simulink library "lib_controller"  (R2015a)
settings: Solver=ode45  StartTime=0.0  StopTime=10.0  RelTol=1e-3
values from neighbouring files (symbols this model uses):
  CG_0 = [0,0,0.02]'    [SetupComplete.m]
  g = 9.81    [SetupComplete.m]
  h_M = 0.064    [SetupComplete.m]
  I_BAC_0 = [ Ix,0,Ixz;0,Iy,0;Ixz,0,Iz]    [SetupComplete.m]
  l = 0.3450    (= 0.345)    [NDI_components.m]    (also in SetupComplete.m; robust_controller.m)
  m = 3.51    [SetupComplete.m]
  m_0 = 2.61    [SetupComplete.m]
  m_M = 0.300    (= 0.3)    [SetupComplete.m]
  T_sim = 0.01    [Run3Copter.m]
undefined symbols (not defined in the file or in its folder): Theta_1_roll_last, Theta_2_roll_last, Theta_3_roll_last, V_long_lastA_w_z, V_long_lastAoA, V_roll_last, V_yaw_last, W_long_lastA_w_z, W_long_lastAoA, W_roll_last, W_yaw_last
libraries: simulink x65, Adaptive_FaultTolerantControl x8, lib_controller x5, qcatlib x4, dspinverses x4, aerolibtransform2 x3, aerolib6dofsys x1
(part 8 of 10)

== matlab function lib_controller/Controller/NDI+CA Controller/4DOF NDI+CA Controller/F(X)1 ==
  data: I_BAC input; CG input; gx output; prev_input input
function gx = gx(I_BAC, CG, prev_input)
    % Calculates f_hat(x). The expression is calculated in NDI_components
    % x_dot = f(x) + g(x,u)
    %   g(x,u) ~= g(x,u0) + jac(g(x,u), u)(u0) * (u - u0)
    %   g(x,u) ~= h(x,u0) + jac(g(x,u), u)(u0) * u
    % x_dot = f_hat(x) + jac(g(x,u), u) * u
    %   f_hat(x) = f(x) + g(x,u0) - jac(g(x,u), u)(u0) *  u0
    %   g_hat(x) = jac(g(x,u), u)(u0)
    % x_dot = f_hat(x) + g_hat(x) * u
    Ixx = I_BAC(1,1);
    Iyy = I_BAC(2,2);
    Izz = I_BAC(3,3);
    Ixz = I_BAC(1,3);
    Iyz = I_BAC(2,3);
    cx = CG(1);
    cy = CG(2);
    cz = CG(3);
    tau1_0 = prev_input(1);
    eta1_0 = prev_input(2);
    gamma1_0 = prev_input(3);
    tau2_0 = prev_input(4);
    eta2_0 = prev_input(5);
    gamma2_0 = prev_input(6);
    tau3_0 = prev_input(7);
    eta3_0 = prev_input(8);
    gamma3_0 = prev_input(9);

 gx = [...
     
                                                                                                                                                                                                                                                                                                                                                         (Gx*Ixx*Iyz^2 + Gx*Ixz^2*Iyy + Gx*Ixy^2*Izz + 2*Gx*Ixy*Ixz*Iyz - Gx*Ixx*Iyy*Izz + Ixy^3*P^2*cy*mass + Ixz^3*P^2*cz*mass - Ixy^3*Q^2*cy*mass - Ixz^3*R^2*cz*mass - Ixx*Iyz^2*Q*W*mass + Ixx*Iyz^2*R*V*mass - Ixz^2*Iyy*Q*W*mass + Ixz^2*Iyy*R*V*mass - Ixy^2*Izz*Q*W*mass + Ixy^2*Izz*R*V*mass + Ixy*Ixz^2*P^2*cy*mass + Ixy^2*Ixz*P^2*cz*mass + Ixx*Iyz^2*Q^2*cx*mass + Ixz^2*Iyy*Q^2*cx*mass - Ixy*Iyz^2*Q^2*cy*mass - Ixy^2*Ixz*Q^2*cz*mass + Ixy^2*Izz*Q^2*cx*mass + Ixz*Iyz^2*Q^2*cz*mass + Ixx*Iyz^2*R^2*cx*mass - Ixy*Ixz^2*R^2*cy*mass + Ixz^2*Iyy*R^2*cx*mass + Ixy*Iyz^2*R^2*cy*mass + Ixy^2*Izz*R^2*cx*mass - Ixz*Iyz^2*R^2*cz*mass + Ixx*Iyz^2*Kt*gamma1_0*tau1_0*cos(gamma1_0) + Ixz^2*Iyy*Kt*gamma1_0*tau1_0*cos(gamma1_0) + Ixy^2*Izz*Kt*gamma1_0*tau1_0*cos(gamma1_0) - 2*Ixy*Ixz*Iyz*Q*W*mass + 2*Ixy*Ixz*Iyz*R*V*mass + Ixx*Iyy*Izz*Q*W*mass - Ixx*Iyy*Izz*R*V*mass - Ixx*Ixy*Iyy*P^2*cy*mass + Ixx*Ixz*Iyz*P^2*cy*mass + Ixx*Ixy*Iyz*P^2*cz*mass - Ixx*Ixz*Izz*P^2*cz*mass + 2*Ixy*Ixz*Iyz*Q^2*cx*mass + Ixx*Ixy*Iyy*Q^2*cy*mass - Ixx*Ixy*Iyz*Q^2*cz*mass - Ixx*Iyy*Izz*Q^2*cx*mass - Ixz*Iyy*Iyz*Q^2*cy*mass + Ixy*Iyz*Izz*Q^2*cz*mass + 2*Ixy*Ixz*Iyz*R^2*cx*mass - Ixx*Ixz*Iyz*R^2*cy*mass - Ixx*Iyy*Izz*R^2*cx*mass + Ixz*Iyy*Iyz*R^2*cy*mass + Ixx*Ixz*Izz*R^2*cz*mass - Ixy*Iyz*Izz*R^2*cz*mass + Ixx*Ixy^2*P*Q*cy*mass + Ixx*Iyy^2*P*Q*cy*mass - Ixx^2*Iyy*P*Q*cy*mass - Ixy^2*Iyy*P*Q*cy*mass - 2*Ixz^2*Iyy*P*Q*cy*mass + Ixx^2*Iyz*P*Q*cz*mass - Ixy^2*Izz*P*Q*cy*mass + 2*Ixz^2*Iyz*P*Q*cz*mass + Ixx*Ixz^2*P*R*cz*mass + Ixx^2*Iyz*P*R*cy*mass + 2*Ixy^2*Iyz*P*R*cy*mass - Ixz^2*Iyy*P*R*cz*mass + Ixx*Izz^2*P*R*cz*mass - Ixx^2*Izz*P*R*cz*mass - 2*Ixy^2*Izz*P*R*cz*mass - Ixz^2*Izz*P*R*cz*mass - 2*Ixy^2*Ixz*Q*R*cy*mass - 2*Ixy*Ixz^2*Q*R*cz*mass - Ixz*Iyy^2*Q*R*cy*mass - Ixy*Izz^2*Q*R*cz*mass + Ixx*Iyz^2*Kt*eta2_0*tau2_0*cos(eta2_0)*cos(gamma2_0) + Ixx*Iyz^2*Kt*eta3_0*tau3_0*cos(eta3_0)*cos(gamma3_0) + Ixz^2*Iyy*Kt*eta2_0*tau2_0*cos(eta2_0)*cos(gamma2_0) + Ixz^2*Iyy*Kt*eta3_0*tau3_0*cos(eta3_0)*cos(gamma3_0) + Ixy^2*Izz*Kt*eta2_0*tau2_0*cos(eta2_0)*cos(gamma2_0) + Ixy^2*Izz*Kt*eta3_0*tau3_0*cos(eta3_0)*cos(gamma3_0) - Ixx*Iyz^2*Kt*gamma2_0*tau2_0*sin(eta2_0)*sin(gamma2_0) - Ixx*Iyz^2*Kt*gamma3_0*tau3_0*sin(eta3_0)*sin(gamma3_0) - Ixz^2*Iyy*Kt*gamma2_0*tau2_0*sin(eta2_0)*sin(gamma2_0) - Ixz^2*Iyy*Kt*gamma3_0*tau3_0*sin(eta3_0)*sin(gamma3_0) - Ixy^2*Izz*Kt*gamma2_0*tau2_0*sin(eta2_0)*sin(gamma2_0) - Ixy^2*Izz*Kt*gamma3_0*tau3_0*sin(eta3_0)*sin(gamma3_0) + 2*Ixy*Ixz*Iyz*Kt*gamma1_0*tau1_0*cos(gamma1_0) - Ixx*Iyy*Izz*Kt*gamma1_0*tau1_0*cos(gamma1_0) + Ixx*Ixy*Ixz*P*Q*cz*mass - 2*Ixy*Ixz*Iyz*P*Q*cy*mass - Ixy*Ixz*Iyy*P*Q*cz*mass - Ixx*Iyy*Iyz*P*Q*cz*mass + Ixx*Iyy*Izz*P*Q*cy*mass + Ixy*Ixz*Izz*P*Q*cz*mass - Ixx*Iyz*Izz*P*Q*cz*mass + Ixx*Ixy*Ixz*P*R*cy*mass + Ixy*Ixz*Iyy*P*R*cy*mass - Ixx*Iyy*Iyz*P*R*cy*mass - 2*Ixy*Ixz*Iyz*P*R*cz*mass - Ixy*Ixz*Izz*P*R*cy*mass - Ixx*Iyz*Izz*P*R*cy*mass + Ixx*Iyy*Izz*P*R*cz*mass - Ixx*Ixy*Iyz*Q*R*cy*mass + Ixx*Ixz*Iyy*Q*R*cy*mass - Ixx*Ixz*Iyz*Q*R*cz*mass - Ixy*Iyy*Iyz*Q*R*cy*mass + Ixx*Ixy*Izz*Q*R*cz*mass + Ixy*Iyz*Izz*Q*R*cy*mass + Ixz*Iyy*Iyz*Q*R*cz*mass + Ixz*Iyy*Izz*Q*R*cy*mass + Ixy*Iyy*Izz*Q*R*cz*mass - Ixz*Iyz*Izz*Q*R*cz*mass - Ixz^2*Kq*cz*gamma2_0*mass*tau2_0*cos(gamma2_0) - Ixz^2*Kq*cz*gamma3_0*mass*tau3_0*cos(gamma3_0) - 2*Ixy*Ixz*Iyz*Kt*gamma2_0*tau2_0*sin(eta2_0)*sin(gamma2_0) - 2*Ixy*Ixz*Iyz*Kt*gamma3_0*tau3_0*sin(eta3_0)*sin(gamma3_0) + Ixx*Iyy*Izz*Kt*gamma2_0*tau2_0*sin(eta2_0)*sin(gamma2_0) + Ixx*Iyy*Izz*Kt*gamma3_0*tau3_0*sin(eta3_0)*sin(gamma3_0) + Ixz^2*Kq*cz*eta1_0*mass*tau1_0*cos(eta1_0)*cos(gamma1_0) - Ixy^2*Kq*cy*eta1_0*mass*tau1_0*cos(gamma1_0)*sin(eta1_0) + Ixy^2*Kq*cy*eta2_0*mass*tau2_0*cos(gamma2_0)*sin(eta2_0) + Ixy^2*Kq*cy*eta3_0*mass*tau3_0*cos(gamma3_0)*sin(eta3_0) - Ixy^2*Kq*cy*gamma1_0*mass*tau1_0*cos(eta1_0)*sin(gamma1_0) + Ixy^2*Kq*cy*gamma2_0*mass*tau2_0*cos(eta2_0)*sin(gamma2_0) + Ixy^2*Kq*cy*gamma3_0*mass*tau3_0*cos(eta3_0)*sin(gamma3_0) - Ixz^2*Kq*cz*gamma1_0*mass*tau1_0*sin(eta1_0)*sin(gamma1_0) - Ixy*Ixz*Kq*cy*gamma2_0*mass*tau2_0*cos(gamma2_0) - Ixy*Ixz*Kq*cy*gamma3_0*mass*tau3_0*cos(gamma3_0) - Ixx*Iyz*Kq*cy*gamma2_0*mass*tau2_0*cos(gamma2_0) - Ixx*Iyz*Kq*cy*gamma3_0*mass*tau3_0*cos(gamma3_0) - Ixy*Iyz*Kq*cy*gamma1_0*mass*tau1_0*cos(gamma1_0) - Ixz*Iyy*Kq*cy*gamma1_0*mass*tau1_0*cos(gamma1_0) + Ixz*Iyz*Kq*cz*gamma1_0*mass*tau1_0*cos(gamma1_0) + Ixx*Izz*Kq*cz*gamma2_0*mass*tau2_0*cos(gamma2_0) + Ixx*Izz*Kq*cz*gamma3_0*mass*tau3_0*cos(gamma3_0) + Ixy*Izz*Kq*cz*gamma1_0*mass*tau1_0*cos(gamma1_0) + 2*Ixy*Ixz*Iyz*Kt*eta2_0*tau2_0*cos(eta2_0)*cos(gamma2_0) + 2*Ixy*Ixz*Iyz*Kt*eta3_0*tau3_0*cos(eta3_0)*cos(gamma3_0) - Ixx*Iyy*Izz*Kt*eta2_0*tau2_0*cos(eta2_0)*cos(gamma2_0) - Ixx*Iyy*Izz*Kt*eta3_0*tau3_0*cos(eta3_0)*cos(gamma3_0) + Ixy*Ixz*Kq*cy*eta1_0*mass*tau1_0*cos(eta1_0)*cos(gamma1_0) + Ixx*Iyz*Kq*cy*eta1_0*mass*tau1_0*cos(eta1_0)*cos(gamma1_0) + Ixy*Iyz*Kq*cy*eta2_0*mass*tau2_0*cos(eta2_0)*cos(gamma2_0) + Ixz*Iyy*Kq*cy*eta2_0*mass*tau2_0*cos(eta2_0)*cos(gamma2_0) + Ixy*Iyz*Kq*cy*eta3_0*mass*tau3_0*cos(eta3_0)*cos(gamma3_0) + Ixz*Iyy*Kq*cy*eta3_0*mass*tau3_0*cos(eta3_0)*cos(gamma3_0) - Ixz*Iyz*Kq*cz*eta2_0*mass*tau2_0*cos(eta2_0)*cos(gamma2_0) - Ixz*Iyz*Kq*cz*eta3_0*mass*tau3_0*cos(eta3_0)*cos(gamma3_0) - Ixx*Izz*Kq*cz*eta1_0*mass*tau1_0*cos(eta1_0)*cos(gamma1_0) - Ixy*Izz*Kq*cz*eta2_0*mass*tau2_0*cos(eta2_0)*cos(gamma2_0) - Ixy*Izz*Kq*cz*eta3_0*mass*tau3_0*cos(eta3_0)*cos(gamma3_0) + Ixx*Iyy*Kq*cy*eta1_0*mass*tau1_0*cos(gamma1_0)*sin(eta1_0) - Ixx*Iyy*Kq*cy*eta2_0*mass*tau2_0*cos(gamma2_0)*sin(eta2_0) - Ixx*Iyy*Kq*cy*eta3_0*mass*tau3_0*cos(gamma3_0)*sin(eta3_0) - Ixy*Ixz*Kq*cz*eta1_0*mass*tau1_0*cos(gamma1_0)*sin(eta1_0) + Ixy*Ixz*Kq*cz*eta2_0*mass*tau2_0*cos(gamma2_0)*sin(eta2_0) + Ixy*Ixz*Kq*cz*eta3_0*mass*tau3_0*cos(gamma3_0)*sin(eta3_0) - Ixx*Iyz*Kq*cz*eta1_0*mass*tau1_0*cos(gamma1_0)*sin(eta1_0) + Ixx*Iyz*Kq*cz*eta2_0*mass*tau2_0*cos(gamma2_0)*sin(eta2_0) + Ixx*Iyz*Kq*cz*eta3_0*mass*tau3_0*cos(gamma3_0)*sin(eta3_0) + Ixx*Iyy*Kq*cy*gamma1_0*mass*tau1_0*cos(eta1_0)*sin(gamma1_0) - Ixx*Iyy*Kq*cy*gamma2_0*mass*tau2_0*cos(eta2_0)*sin(gamma2_0) - Ixx*Iyy*Kq*cy*gamma3_0*mass*tau3_0*cos(eta3_0)*sin(gamma3_0) - Ixy*Ixz*Kq*cz*gamma1_0*mass*tau1_0*cos(eta1_0)*sin(gamma1_0) + Ixy*Ixz*Kq*cz*gamma2_0*mass*tau2_0*cos(eta2_0)*sin(gamma2_0) + Ixy*Ixz*Kq*cz*gamma3_0*mass*tau3_0*cos(eta3_0)*sin(gamma3_0) - Ixx*Iyz*Kq*cz*gamma1_0*mass*tau1_0*cos(eta1_0)*sin(gamma1_0) + Ixx*Iyz*Kq*cz*gamma2_0*mass*tau2_0*cos(eta2_0)*sin(gamma2_0) + Ixx*Iyz*Kq*cz*gamma3_0*mass*tau3_0*cos(eta3_0)*sin(gamma3_0) - Ixy*Ixz*Kq*cy*gamma1_0*mass*tau1_0*sin(eta1_0)*sin(gamma1_0) - Ixx*Iyz*Kq*cy*gamma1_0*mass*tau1_0*sin(eta1_0)*sin(gamma1_0) - Ixy*Iyz*Kq*cy*gamma2_0*mass*tau2_0*sin(eta2_0)*sin(gamma2_0) - Ixz*Iyy*Kq*cy*gamma2_0*mass*tau2_0*sin(eta2_0)*sin(gamma2_0) - Ixy*Iyz*Kq*cy*gamma3_0*mass*tau3_0*sin(eta3_0)*sin(gamma3_0) - Ixz*Iyy*Kq*cy*gamma3_0*mass*tau3_0*sin(eta3_0)*sin(gamma3_0) + Ixz*Iyz*Kq*cz*gamma2_0*mass*tau2_0*sin(eta2_0)*sin(gamma2_0) + Ixz*Iyz*Kq*cz*gamma3_0*mass*tau3_0*sin(eta3_0)*sin(gamma3_0) + Ixx*Izz*Kq*cz*gamma1_0*mass*tau1_0*sin(eta1_0)*sin(gamma1_0) + Ixy*Izz*Kq*cz*gamma2_0*mass*tau2_0*sin(eta2_0)*sin(gamma2_0) + Ixy*Izz*Kq*cz*gamma3_0*mass*tau3_0*sin(eta3_0)*sin(gamma3_0))/(mass*(Izz*Ixy^2 + 2*Ixy*Ixz*Iyz + Iyy*Ixz^2 + Ixx*Iyz^2 - Ixx*Iyy*Izz));
                                                                                                                                                                                                                                                                                                                                                                                                                                                                                                                                                                                                                                                                                                               -(Gy*Ixx*Iyy*Izz - Gy*Ixz^2*Iyy - Gy*Ixy^2*Izz - 2*Gy*Ixy*Ixz*Iyz - Gy*Ixx*Iyz^2 + Ixy^3*P^2*cx*mass - Ixy^3*Q^2*cx*mass - Iyz^3*Q^2*cz*mass + Iyz^3*R^2*cz*mass - Ixx*Iyz^2*P*W*mass + Ixx*Iyz^2*R*U*mass - Ixz^2*Iyy*P*W*mass + Ixz^2*Iyy*R*U*mass - Ixy^2*Izz*P*W*mass + Ixy^2*Izz*R*U*mass + Ixy*Ixz^2*P^2*cx*mass - Ixx*Iyz^2*P^2*cy*mass - Ixz^2*Iyy*P^2*cy*mass + Ixy^2*Iyz*P^2*cz*mass - Ixy^2*Izz*P^2*cy*mass - Ixz^2*Iyz*P^2*cz*mass - Ixy*Iyz^2*Q^2*cx*mass - Ixy^2*Iyz*Q^2*cz*mass - Ixy*Ixz^2*R^2*cx*mass + Ixy*Iyz^2*R^2*cx*mass - Ixx*Iyz^2*R^2*cy*mass - Ixz^2*Iyy*R^2*cy*mass - Ixy^2*Izz*R^2*cy*mass + Ixz^2*Iyz*R^2*cz*mass + Ixx*Iyz^2*Kt*gamma2_0*tau2_0*cos(gamma2_0) + Ixx*Iyz^2*Kt*gamma3_0*tau3_0*cos(gamma3_0) + Ixz^2*Iyy*Kt*gamma2_0*tau2_0*cos(gamma2_0) + Ixz^2*Iyy*Kt*gamma3_0*tau3_0*cos(gamma3_0) + Ixy^2*Izz*Kt*gamma2_0*tau2_0*cos(gamma2_0) + Ixy^2*Izz*Kt*gamma3_0*tau3_0*cos(gamma3_0) - 2*Ixy*Ixz*Iyz*P*W*mass + 2*Ixy*Ixz*Iyz*R*U*mass + Ixx*Iyy*Izz*P*W*mass - Ixx*Iyy*Izz*R*U*mass - Ixx*Ixy*Iyy*P^2*cx*mass + Ixx*Ixz*Iyz*P^2*cx*mass - 2*Ixy*Ixz*Iyz*P^2*cy*mass + Ixy*Ixz*Iyy*P^2*cz*mass + Ixx*Iyy*Izz*P^2*cy*mass - Ixy*Ixz*Izz*P^2*cz*mass + Ixx*Ixy*Iyy*Q^2*cx*mass - Ixz*Iyy*Iyz*Q^2*cx*mass - Ixy*Ixz*Iyy*Q^2*cz*mass + Iyy*Iyz*Izz*Q^2*cz*mass - Ixx*Ixz*Iyz*R^2*cx*mass - 2*Ixy*Ixz*Iyz*R^2*cy*mass + Ixz*Iyy*Iyz*R^2*cx*mass + Ixx*Iyy*Izz*R^2*cy*mass + Ixy*Ixz*Izz*R^2*cz*mass - Iyy*Iyz*Izz*R^2*cz*mass + Ixx*Ixy^2*P*Q*cx*mass + Ixx*Iyy^2*P*Q*cx*mass - Ixx^2*Iyy*P*Q*cx*mass + 2*Ixx*Iyz^2*P*Q*cx*mass - Ixy^2*Iyy*P*Q*cx*mass + Ixy^2*Izz*P*Q*cx*mass - Ixz*Iyy^2*P*Q*cz*mass - 2*Ixz*Iyz^2*P*Q*cz*mass + Ixx^2*Iyz*P*R*cx*mass + 2*Ixy^2*Iyz*P*R*cx*mass + 2*Ixy*Iyz^2*P*R*cz*mass + Ixy*Izz^2*P*R*cz*mass - 2*Ixy^2*Ixz*Q*R*cx*mass - Ixz*Iyy^2*Q*R*cx*mass + Ixx*Iyz^2*Q*R*cz*mass - Iyy*Iyz^2*Q*R*cz*mass + 2*Ixy^2*Izz*Q*R*cz*mass - Iyy*Izz^2*Q*R*cz*mass + Iyy^2*Izz*Q*R*cz*mass + Iyz^2*Izz*Q*R*cz*mass + Ixx*Iyz^2*Kt*eta1_0*tau1_0*cos(eta1_0)*cos(gamma1_0) + Ixz^2*Iyy*Kt*eta1_0*tau1_0*cos(eta1_0)*cos(gamma1_0) + Ixy^2*Izz*Kt*eta1_0*tau1_0*cos(eta1_0)*cos(gamma1_0) - Ixx*Iyz^2*Kt*gamma1_0*tau1_0*sin(eta1_0)*sin(gamma1_0) - Ixz^2*Iyy*Kt*gamma1_0*tau1_0*sin(eta1_0)*sin(gamma1_0) - Ixy^2*Izz*Kt*gamma1_0*tau1_0*sin(eta1_0)*sin(gamma1_0) + 2*Ixy*Ixz*Iyz*Kt*gamma2_0*tau2_0*cos(gamma2_0) + 2*Ixy*Ixz*Iyz*Kt*gamma3_0*tau3_0*cos(gamma3_0) - Ixx*Iyy*Izz*Kt*gamma2_0*tau2_0*cos(gamma2_0) - Ixx*Iyy*Izz*Kt*gamma3_0*tau3_0*cos(gamma3_0) + 2*Ixy*Ixz*Iyz*P*Q*cx*mass + Ixx*Ixy*Iyz*P*Q*cz*mass + Ixx*Ixz*Iyy*P*Q*cz*mass - Ixx*Iyy*Izz*P*Q*cx*mass - Ixy*Iyy*Iyz*P*Q*cz*mass - Ixy*Iyz*Izz*P*Q*cz*mass + Ixz*Iyy*Izz*P*Q*cz*mass + Ixx*Ixy*Ixz*P*R*cx*mass + Ixy*Ixz*Iyy*P*R*cx*mass - Ixx*Iyy*Iyz*P*R*cx*mass - Ixy*Ixz*Izz*P*R*cx*mass - Ixx*Ixz*Iyz*P*R*cz*mass - Ixx*Iyz*Izz*P*R*cx*mass - Ixx*Ixy*Izz*P*R*cz*mass + Ixz*Iyy*Iyz*P*R*cz*mass - Ixy*Iyy*Izz*P*R*cz*mass + Ixz*Iyz*Izz*P*R*cz*mass - Ixx*Ixy*Iyz*Q*R*cx*mass + Ixx*Ixz*Iyy*Q*R*cx*mass - Ixy*Iyy*Iyz*Q*R*cx*mass + 2*Ixy*Ixz*Iyz*Q*R*cz*mass + Ixy*Iyz*Izz*Q*R*cx*mass + Ixz*Iyy*Izz*Q*R*cx*mass - Ixx*Iyy*Izz*Q*R*cz*mass - Iyz^2*Kq*cz*gamma1_0*mass*tau1_0*cos(gamma1_0) - 2*Ixy*Ixz*Iyz*Kt*gamma1_0*tau1_0*sin(eta1_0)*sin(gamma1_0) + Ixx*Iyy*Izz*Kt*gamma1_0*tau1_0*sin(eta1_0)*sin(gamma1_0) + Iyz^2*Kq*cz*eta2_0*mass*tau2_0*cos(eta2_0)*cos(gamma2_0) + Iyz^2*Kq*cz*eta3_0*mass*tau3_0*cos(eta3_0)*cos(gamma3_0) - Ixy^2*Kq*cx*eta1_0*mass*tau1_0*cos(gamma1_0)*sin(eta1_0) + Ixy^2*Kq*cx*eta2_0*mass*tau2_0*cos(gamma2_0)*sin(eta2_0) + Ixy^2*Kq*cx*eta3_0*mass*tau3_0*cos(gamma3_0)*sin(eta3_0) - Ixy^2*Kq*cx*gamma1_0*mass*tau1_0*cos(eta1_0)*sin(gamma1_0) + Ixy^2*Kq*cx*gamma2_0*mass*tau2_0*cos(eta2_0)*sin(gamma2_0) + Ixy^2*Kq*cx*gamma3_0*mass*tau3_0*cos(eta3_0)*sin(gamma3_0) - Iyz^2*Kq*cz*gamma2_0*mass*tau2_0*sin(eta2_0)*sin(gamma2_0) - Iyz^2*Kq*cz*gamma3_0*mass*tau3_0*sin(eta3_0)*sin(gamma3_0) - Ixy*Ixz*Kq*cx*gamma2_0*mass*tau2_0*cos(gamma2_0) - Ixy*Ixz*Kq*cx*gamma3_0*mass*tau3_0*cos(gamma3_0) - Ixx*Iyz*Kq*cx*gamma2_0*mass*tau2_0*cos(gamma2_0) - Ixx*Iyz*Kq*cx*gamma3_0*mass*tau3_0*cos(gamma3_0) - Ixy*Iyz*Kq*cx*gamma1_0*mass*tau1_0*cos(gamma1_0) - Ixz*Iyy*Kq*cx*gamma1_0*mass*tau1_0*cos(gamma1_0) + Ixz*Iyz*Kq*cz*gamma2_0*mass*tau2_0*cos(gamma2_0) + Ixz*Iyz*Kq*cz*gamma3_0*mass*tau3_0*cos(gamma3_0) + Ixy*Izz*Kq*cz*gamma2_0*mass*tau2_0*cos(gamma2_0) + Ixy*Izz*Kq*cz*gamma3_0*mass*tau3_0*cos(gamma3_0) + Iyy*Izz*Kq*cz*gamma1_0*mass*tau1_0*cos(gamma1_0) + 2*Ixy*Ixz*Iyz*Kt*eta1_0*tau1_0*cos(eta1_0)*cos(gamma1_0) - Ixx*Iyy*Izz*Kt*eta1_0*tau1_0*cos(eta1_0)*cos(gamma1_0) + Ixy*Ixz*Kq*cx*eta1_0*mass*tau1_0*cos(eta1_0)*cos(gamma1_0) + Ixx*Iyz*Kq*cx*eta1_0*mass*tau1_0*cos(eta1_0)*cos(gamma1_0) + Ixy*Iyz*Kq*cx*eta2_0*mass*tau2_0*cos(eta2_0)*cos(gamma2_0) + Ixz*Iyy*Kq*cx*eta2_0*mass*tau2_0*cos(eta2_0)*cos(gamma2_0) + Ixy*Iyz*Kq*cx*eta3_0*mass*tau3_0*cos(eta3_0)*cos(gamma3_0) + Ixz*Iyy*Kq*cx*eta3_0*mass*tau3_0*cos(eta3_0)*cos(gamma3_0) - Ixz*Iyz*Kq*cz*eta1_0*mass*tau1_0*cos(eta1_0)*cos(gamma1_0) - Ixy*Izz*Kq*cz*eta1_0*mass*tau1_0*cos(eta1_0)*cos(gamma1_0) - Iyy*Izz*Kq*cz*eta2_0*mass*tau2_0*cos(eta2_0)*cos(gamma2_0) - Iyy*Izz*Kq*cz*eta3_0*mass*tau3_0*cos(eta3_0)*cos(gamma3_0) + Ixx*Iyy*Kq*cx*eta1_0*mass*tau1_0*cos(gamma1_0)*sin(eta1_0) - Ixx*Iyy*Kq*cx*eta2_0*mass*tau2_0*cos(gamma2_0)*sin(eta2_0) - Ixx*Iyy*Kq*cx*eta3_0*mass*tau3_0*cos(gamma3_0)*sin(eta3_0) - Ixy*Iyz*Kq*cz*eta1_0*mass*tau1_0*cos(gamma1_0)*sin(eta1_0) - Ixz*Iyy*Kq*cz*eta1_0*mass*tau1_0*cos(gamma1_0)*sin(eta1_0) + Ixy*Iyz*Kq*cz*eta2_0*mass*tau2_0*cos(gamma2_0)*sin(eta2_0) + Ixz*Iyy*Kq*cz*eta2_0*mass*tau2_0*cos(gamma2_0)*sin(eta2_0) + Ixy*Iyz*Kq*cz*eta3_0*mass*tau3_0*cos(gamma3_0)*sin(eta3_0) + Ixz*Iyy*Kq*cz*eta3_0*mass*tau3_0*cos(gamma3_0)*sin(eta3_0) + Ixx*Iyy*Kq*cx*gamma1_0*mass*tau1_0*cos(eta1_0)*sin(gamma1_0) - Ixx*Iyy*Kq*cx*gamma2_0*mass*tau2_0*cos(eta2_0)*sin(gamma2_0) - Ixx*Iyy*Kq*cx*gamma3_0*mass*tau3_0*cos(eta3_0)*sin(gamma3_0) - Ixy*Iyz*Kq*cz*gamma1_0*mass*tau1_0*cos(eta1_0)*sin(gamma1_0) - Ixz*Iyy*Kq*cz*gamma1_0*mass*tau1_0*cos(eta1_0)*sin(gamma1_0) + Ixy*Iyz*Kq*cz*gamma2_0*mass*tau2_0*cos(eta2_0)*sin(gamma2_0) + Ixz*Iyy*Kq*cz*gamma2_0*mass*tau2_0*cos(eta2_0)*sin(gamma2_0) + Ixy*Iyz*Kq*cz*gamma3_0*mass*tau3_0*cos(eta3_0)*sin(gamma3_0) + Ixz*Iyy*Kq*cz*gamma3_0*mass*tau3_0*cos(eta3_0)*sin(gamma3_0) - Ixy*Ixz*Kq*cx*gamma1_0*mass*tau1_0*sin(eta1_0)*sin(gamma1_0) - Ixx*Iyz*Kq*cx*gamma1_0*mass*tau1_0*sin(eta1_0)*sin(gamma1_0) - Ixy*Iyz*Kq*cx*gamma2_0*mass*tau2_0*sin(eta2_0)*sin(gamma2_0) - Ixz*Iyy*Kq*cx*gamma2_0*mass*tau2_0*sin(eta2_0)*sin(gamma2_0) - Ixy*Iyz*Kq*cx*gamma3_0*mass*tau3_0*sin(eta3_0)*sin(gamma3_0) - Ixz*Iyy*Kq*cx*gamma3_0*mass*tau3_0*sin(eta3_0)*sin(gamma3_0) + Ixz*Iyz*Kq*cz*gamma1_0*mass*tau1_0*sin(eta1_0)*sin(gamma1_0) + Ixy*Izz*Kq*cz*gamma1_0*mass*tau1_0*sin(eta1_0)*sin(gamma1_0) + Iyy*Izz*Kq*cz*gamma2_0*mass*tau2_0*sin(eta2_0)*sin(gamma2_0) + Iyy*Izz*Kq*cz*gamma3_0*mass*tau3_0*sin(eta3_0)*sin(gamma3_0))/(mass*(Izz*Ixy^2 + 2*Ixy*Ixz*Iyz + Iyy*Ixz^2 + Ixx*Iyz^2 - Ixx*Iyy*Izz));
 -(Gz*Ixx*Iyy*Izz - Gz*Ixz^2*Iyy - Gz*Ixy^2*Izz - 2*Gz*Ixy*Ixz*Iyz - Gz*Ixx*Iyz^2 + Ixz^3*P^2*cx*mass + Iyz^3*Q^2*cy*mass - Ixz^3*R^2*cx*mass - Iyz^3*R^2*cy*mass + Ixx*Iyz^2*P*V*mass - Ixx*Iyz^2*Q*U*mass + Ixz^2*Iyy*P*V*mass - Ixz^2*Iyy*Q*U*mass + Ixy^2*Izz*P*V*mass - Ixy^2*Izz*Q*U*mass + Ixy^2*Ixz*P^2*cx*mass - Ixy^2*Iyz*P^2*cy*mass + Ixz^2*Iyz*P^2*cy*mass - Ixx*Iyz^2*P^2*cz*mass - Ixz^2*Iyy*P^2*cz*mass - Ixy^2*Izz*P^2*cz*mass - Ixy^2*Ixz*Q^2*cx*mass + Ixz*Iyz^2*Q^2*cx*mass + Ixy^2*Iyz*Q^2*cy*mass - Ixx*Iyz^2*Q^2*cz*mass - Ixz^2*Iyy*Q^2*cz*mass - Ixy^2*Izz*Q^2*cz*mass - Ixz*Iyz^2*R^2*cx*mass - Ixz^2*Iyz*R^2*cy*mass + 2*Ixy*Ixz*Iyz*P*V*mass - 2*Ixy*Ixz*Iyz*Q*U*mass - Ixx*Iyy*Izz*P*V*mass + Ixx*Iyy*Izz*Q*U*mass + Ixx*Ixy*Iyz*P^2*cx*mass - Ixx*Ixz*Izz*P^2*cx*mass - Ixy*Ixz*Iyy*P^2*cy*mass - 2*Ixy*Ixz*Iyz*P^2*cz*mass + Ixy*Ixz*Izz*P^2*cy*mass + Ixx*Iyy*Izz*P^2*cz*mass - Ixx*Ixy*Iyz*Q^2*cx*mass + Ixy*Ixz*Iyy*Q^2*cy*mass - 2*Ixy*Ixz*Iyz*Q^2*cz*mass + Ixy*Iyz*Izz*Q^2*cx*mass + Ixx*Iyy*Izz*Q^2*cz*mass - Iyy*Iyz*Izz*Q^2*cy*mass + Ixx*Ixz*Izz*R^2*cx*mass - Ixy*Ixz*Izz*R^2*cy*mass - Ixy*Iyz*Izz*R^2*cx*mass + Iyy*Iyz*Izz*R^2*cy*mass + Ixx^2*Iyz*P*Q*cx*mass + 2*Ixz^2*Iyz*P*Q*cx*mass + Ixz*Iyy^2*P*Q*cy*mass + 2*Ixz*Iyz^2*P*Q*cy*mass + Ixx*Ixz^2*P*R*cx*mass + 2*Ixx*Iyz^2*P*R*cx*mass + Ixz^2*Iyy*P*R*cx*mass + Ixx*Izz^2*P*R*cx*mass - Ixx^2*Izz*P*R*cx*mass - 2*Ixy*Iyz^2*P*R*cy*mass - Ixz^2*Izz*P*R*cx*mass - Ixy*Izz^2*P*R*cy*mass - 2*Ixy*Ixz^2*Q*R*cx*mass + Ixx*Iyz^2*Q*R*cy*mass - Ixy*Izz^2*Q*R*cx*mass + 2*Ixz^2*Iyy*Q*R*cy*mass + Iyy*Iyz^2*Q*R*cy*mass + Iyy*Izz^2*Q*R*cy*mass - Iyy^2*Izz*Q*R*cy*mass - Iyz^2*Izz*Q*R*cy*mass + Ixx*Iyz^2*Kt*eta1_0*tau1_0*cos(gamma1_0)*sin(eta1_0) + Ixx*Iyz^2*Kt*eta2_0*tau2_0*cos(gamma2_0)*sin(eta2_0) + Ixx*Iyz^2*Kt*eta3_0*tau3_0*cos(gamma3_0)*sin(eta3_0) + Ixz^2*Iyy*Kt*eta1_0*tau1_0*cos(gamma1_0)*sin(eta1_0) + Ixz^2*Iyy*Kt*eta2_0*tau2_0*cos(gamma2_0)*sin(eta2_0) + Ixz^2*Iyy*Kt*eta3_0*tau3_0*cos(gamma3_0)*sin(eta3_0) + Ixy^2*Izz*Kt*eta1_0*tau1_0*cos(gamma1_0)*sin(eta1_0) + Ixy^2*Izz*Kt*eta2_0*tau2_0*cos(gamma2_0)*sin(eta2_0) + Ixy^2*Izz*Kt*eta3_0*tau3_0*cos(gamma3_0)*sin(eta3_0) + Ixx*Iyz^2*Kt*gamma1_0*tau1_0*cos(eta1_0)*sin(gamma1_0) + Ixx*Iyz^2*Kt*gamma2_0*tau2_0*cos(eta2_0)*sin(gamma2_0) + Ixx*Iyz^2*Kt*gamma3_0*tau3_0*cos(eta3_0)*sin(gamma3_0) + Ixz^2*Iyy*Kt*gamma1_0*tau1_0*cos(eta1_0)*sin(gamma1_0) + Ixz^2*Iyy*Kt*gamma2_0*tau2_0*cos(eta2_0)*sin(gamma2_0) + Ixz^2*Iyy*Kt*gamma3_0*tau3_0*cos(eta3_0)*sin(gamma3_0) + Ixy^2*Izz*Kt*gamma1_0*tau1_0*cos(eta1_0)*sin(gamma1_0) + Ixy^2*Izz*Kt*gamma2_0*tau2_0*cos(eta2_0)*sin(gamma2_0) + Ixy^2*Izz*Kt*gamma3_0*tau3_0*cos(eta3_0)*sin(gamma3_0) + Ixx*Ixy*Ixz*P*Q*cx*mass - Ixy*Ixz*Iyy*P*Q*cx*mass - Ixx*Ixy*Iyz*P*Q*cy*mass - Ixx*Ixz*Iyy*P*Q*cy*mass - Ixx*Iyy*Iyz*P*Q*cx*mass + Ixy*Ixz*Izz*P*Q*cx*mass - Ixx*Iyz*Izz*P*Q*cx*mass + Ixy*Iyy*Iyz*P*Q*cy*mass + Ixy*Iyz*Izz*P*Q*cy*mass - Ixz*Iyy*Izz*P*Q*cy*mass + 2*Ixy*Ixz*Iyz*P*R*cx*mass + Ixx*Ixz*Iyz*P*R*cy*mass + Ixx*Ixy*Izz*P*R*cy*mass - Ixx*Iyy*Izz*P*R*cx*mass - Ixz*Iyy*Iyz*P*R*cy*mass + Ixy*Iyy*Izz*P*R*cy*mass - Ixz*Iyz*Izz*P*R*cy*mass - Ixx*Ixz*Iyz*Q*R*cx*mass + Ixx*Ixy*Izz*Q*R*cx*mass + 2*Ixy*Ixz*Iyz*Q*R*cy*mass + Ixz*Iyy*Iyz*Q*R*cx*mass + Ixy*Iyy*Izz*Q*R*cx*mass - Ixz*Iyz*Izz*Q*R*cx*mass - Ixx*Iyy*Izz*Q*R*cy*mass - Ixz^2*Kq*cx*gamma2_0*mass*tau2_0*cos(gamma2_0) - Ixz^2*Kq*cx*gamma3_0*mass*tau3_0*cos(gamma3_0) + Iyz^2*Kq*cy*gamma1_0*mass*tau1_0*cos(gamma1_0) + 2*Ixy*Ixz*Iyz*Kt*eta1_0*tau1_0*cos(gamma1_0)*sin(eta1_0) + 2*Ixy*Ixz*Iyz*Kt*eta2_0*tau2_0*cos(gamma2_0)*sin(eta2_0) + 2*Ixy*Ixz*Iyz*Kt*eta3_0*tau3_0*cos(gamma3_0)*sin(eta3_0) - Ixx*Iyy*Izz*Kt*eta1_0*tau1_0*cos(gamma1_0)*sin(eta1_0) - Ixx*Iyy*Izz*Kt*eta2_0*tau2_0*cos(gamma2_0)*sin(eta2_0) - Ixx*Iyy*Izz*Kt*eta3_0*tau3_0*cos(gamma3_0)*sin(eta3_0) + 2*Ixy*Ixz*Iyz*Kt*gamma1_0*tau1_0*cos(eta1_0)*sin(gamma1_0) + 2*Ixy*Ixz*Iyz*Kt*gamma2_0*tau2_0*cos(eta2_0)*sin(gamma2_0) + 2*Ixy*Ixz*Iyz*Kt*gamma3_0*tau3_0*cos(eta3_0)*sin(gamma3_0) - Ixx*Iyy*Izz*Kt*gamma1_0*tau1_0*cos(eta1_0)*sin(gamma1_0) - Ixx*Iyy*Izz*Kt*gamma2_0*tau2_0*cos(eta2_0)*sin(gamma2_0) - Ixx*Iyy*Izz*Kt*gamma3_0*tau3_0*cos(eta3_0)*sin(gamma3_0) + Ixz^2*Kq*cx*eta1_0*mass*tau1_0*cos(eta1_0)*cos(gamma1_0) - Iyz^2*Kq*cy*eta2_0*mass*tau2_0*cos(eta2_0)*cos(gamma2_0) - Iyz^2*Kq*cy*eta3_0*mass*tau3_0*cos(eta3_0)*cos(gamma3_0) - Ixz^2*Kq*cx*gamma1_0*mass*tau1_0*sin(eta1_0)*sin(gamma1_0) + Iyz^2*Kq*cy*gamma2_0*mass*tau2_0*sin(eta2_0)*sin(gamma2_0) + Iyz^2*Kq*cy*gamma3_0*mass*tau3_0*sin(eta3_0)*sin(gamma3_0) + Ixz*Iyz*Kq*cx*gamma1_0*mass*tau1_0*cos(gamma1_0) + Ixx*Izz*Kq*cx*gamma2_0*mass*tau2_0*cos(gamma2_0) + Ixx*Izz*Kq*cx*gamma3_0*mass*tau3_0*cos(gamma3_0) + Ixy*Izz*Kq*cx*gamma1_0*mass*tau1_0*cos(gamma1_0) - Ixz*Iyz*Kq*cy*gamma2_0*mass*tau2_0*cos(gamma2_0) - Ixz*Iyz*Kq*cy*gamma3_0*mass*tau3_0*cos(gamma3_0) - Ixy*Izz*Kq*cy*gamma2_0*mass*tau2_0*cos(gamma2_0) - Ixy*Izz*Kq*cy*gamma3_0*mass*tau3_0*cos(gamma3_0) - Iyy*Izz*Kq*cy*gamma1_0*mass*tau1_0*cos(gamma1_0) - Ixz*Iyz*Kq*cx*eta2_0*mass*tau2_0*cos(eta2_0)*cos(gamma2_0) - Ixz*Iyz*Kq*cx*eta3_0*mass*tau3_0*cos(eta3_0)*cos(gamma3_0) - Ixx*Izz*Kq*cx*eta1_0*mass*tau1_0*cos(eta1_0)*cos(gamma1_0) - Ixy*Izz*Kq*cx*eta2_0*mass*tau2_0*cos(eta2_0)*cos(gamma2_0) - Ixy*Izz*Kq*cx*eta3_0*mass*tau3_0*cos(eta3_0)*cos(gamma3_0) + Ixz*Iyz*Kq*cy*eta1_0*mass*tau1_0*cos(eta1_0)*cos(gamma1_0) + Ixy*Izz*Kq*cy*eta1_0*mass*tau1_0*cos(eta1_0)*cos(gamma1_0) + Iyy*Izz*Kq*cy*eta2_0*mass*tau2_0*cos(eta2_0)*cos(gamma2_0) + Iyy*Izz*Kq*cy*eta3_0*mass*tau3_0*cos(eta3_0)*cos(gamma3_0) - Ixy*Ixz*Kq*cx*eta1_0*mass*tau1_0*cos(gamma1_0)*sin(eta1_0) + Ixy*Ixz*Kq*cx*eta2_0*mass*tau2_0*cos(gamma2_0)*sin(eta2_0) + Ixy*Ixz*Kq*cx*eta3_0*mass*tau3_0*cos(gamma3_0)*sin(eta3_0) - Ixx*Iyz*Kq*cx*eta1_0*mass*tau1_0*cos(gamma1_0)*sin(eta1_0) + Ixx*Iyz*Kq*cx*eta2_0*mass*tau2_0*cos(gamma2_0)*sin(eta2_0) + Ixx*Iyz*Kq*cx*eta3_0*mass*tau3_0*cos(gamma3_0)*sin(eta3_0) + Ixy*Iyz*Kq*cy*eta1_0*mass*tau1_0*cos(gamma1_0)*sin(eta1_0) + Ixz*Iyy*Kq*cy*eta1_0*mass*tau1_0*cos(gamma1_0)*sin(eta1_0) - Ixy*Iyz*Kq*cy*eta2_0*mass*tau2_0*cos(gamma2_0)*sin(eta2_0) - Ixz*Iyy*Kq*cy*eta2_0*mass*tau2_0*cos(gamma2_0)*sin(eta2_0) - Ixy*Iyz*Kq*cy*eta3_0*mass*tau3_0*cos(gamma3_0)*sin(eta3_0) - Ixz*Iyy*Kq*cy*eta3_0*mass*tau3_0*cos(gamma3_0)*sin(eta3_0) - Ixy*Ixz*Kq*cx*gamma1_0*mass*tau1_0*cos(eta1_0)*sin(gamma1_0) + Ixy*Ixz*Kq*cx*gamma2_0*mass*tau2_0*cos(eta2_0)*sin(gamma2_0) + Ixy*Ixz*Kq*cx*gamma3_0*mass*tau3_0*cos(eta3_0)*sin(gamma3_0) - Ixx*Iyz*Kq*cx*gamma1_0*mass*tau1_0*cos(eta1_0)*sin(gamma1_0) + Ixx*Iyz*Kq*cx*gamma2_0*mass*tau2_0*cos(eta2_0)*sin(gamma2_0) + Ixx*Iyz*Kq*cx*gamma3_0*mass*tau3_0*cos(eta3_0)*sin(gamma3_0) + Ixy*Iyz*Kq*cy*gamma1_0*mass*tau1_0*cos(eta1_0)*sin(gamma1_0) + Ixz*Iyy*Kq*cy*gamma1_0*mass*tau1_0*cos(eta1_0)*sin(gamma1_0) - Ixy*Iyz*Kq*cy*gamma2_0*mass*tau2_0*cos(eta2_0)*sin(gamma2_0) - Ixz*Iyy*Kq*cy*gamma2_0*mass*tau2_0*cos(eta2_0)*sin(gamma2_0) - Ixy*Iyz*Kq*cy*gamma3_0*mass*tau3_0*cos(eta3_0)*sin(gamma3_0) - Ixz*Iyy*Kq*cy*gamma3_0*mass*tau3_0*cos(eta3_0)*sin(gamma3_0) + Ixz*Iyz*Kq*cx*gamma2_0*mass*tau2_0*sin(eta2_0)*sin(gamma2_0) + Ixz*Iyz*Kq*cx*gamma3_0*mass*tau3_0*sin(eta3_0)*sin(gamma3_0) + Ixx*Izz*Kq*cx*gamma1_0*mass*tau1_0*sin(eta1_0)*sin(gamma1_0) + Ixy*Izz*Kq*cx*gamma2_0*mass*tau2_0*sin(eta2_0)*sin(gamma2_0) + Ixy*Izz*Kq*cx*gamma3_0*mass*tau3_0*sin(eta3_0)*sin(gamma3_0) - Ixz*Iyz*Kq*cy*gamma1_0*mass*tau1_0*sin(eta1_0)*sin(gamma1_0) - Ixy*Izz*Kq*cy*gamma1_0*mass*tau1_0*sin(eta1_0)*sin(gamma1_0) - Iyy*Izz*Kq*cy*gamma2_0*mass*tau2_0*sin(eta2_0)*sin(gamma2_0) - Iyy*Izz*Kq*cy*gamma3_0*mass*tau3_0*sin(eta3_0)*sin(gamma3_0))/(mass*(Izz*Ixy^2 + 2*Ixy*Ixz*Iyz + Iyy*Ixz^2 + Ixx*Iyz^2 - Ixx*Iyy*Izz));
                                                                                                                                                                                                                                                                                                                                                                                                                                                                                                                                                                                                                                                                                                                                                                                                                                                                                                                                                                                                                                                                                                                                                                                                                                                                                                                                                                                                                                                                                                                                                                                                                                                                                                                                                                                                                                                                                                                                                                                                                                                                                                                                                                                                                                                                                                                                                                                                                                                                                                                                                                                                                                                                                                                                                                                                                                                                                                                                                                                                                                                                                                                                                                                                                                                                                                                                                                                                                                                                                                                                                                                                                                                                                                                                                                                                                                                                                                                                                                                                                                                                                                                                                                                                                                                                                                                                                                                                                                                                                                                                                                                                                                                                                                                                                                                                                                                                                                                                                                                                                                                                                                                                                                                                                                                                                                                                                                                                                                                                                                                                                                                                                                                                                             -(Iyz^3*R^2 - Iyz^3*Q^2 + Ixy^2*Iyz*P^2 - Ixz^2*Iyz*P^2 - Ixy^2*Iyz*Q^2 + Ixz^2*Iyz*R^2 + Ixy*Ixz*Iyy*P^2 - Ixy*Ixz*Izz*P^2 - Ixy*Ixz*Iyy*Q^2 + Iyy*Iyz*Izz*Q^2 + Ixy*Ixz*Izz*R^2 - Iyy*Iyz*Izz*R^2 - Ixz*Iyy^2*P*Q - 2*Ixz*Iyz^2*P*Q + 2*Ixy*Iyz^2*P*R + Ixy*Izz^2*P*R - Ixz^2*Iyy*Q*R - Iyy*Iyz^2*Q*R + Ixy^2*Izz*Q*R - Iyy*Izz^2*Q*R + Iyy^2*Izz*Q*R + Iyz^2*Izz*Q*R + Ixx*Ixy*Iyz*P*Q + Ixx*Ixz*Iyy*P*Q - Ixy*Iyy*Iyz*P*Q - Ixy*Iyz*Izz*P*Q + Ixz*Iyy*Izz*P*Q - Ixx*Ixz*Iyz*P*R - Ixx*Ixy*Izz*P*R + Ixz*Iyy*Iyz*P*R - Ixy*Iyy*Izz*P*R + Ixz*Iyz*Izz*P*R - Iyz^2*Kq*gamma1_0*tau1_0*cos(gamma1_0) + Iyz^2*Kq*eta2_0*tau2_0*cos(eta2_0)*cos(gamma2_0) + Iyz^2*Kq*eta3_0*tau3_0*cos(eta3_0)*cos(gamma3_0) - Iyz^2*Kq*gamma2_0*tau2_0*sin(eta2_0)*sin(gamma2_0) - Iyz^2*Kq*gamma3_0*tau3_0*sin(eta3_0)*sin(gamma3_0) + Ixz*Iyz*Kq*gamma2_0*tau2_0*cos(gamma2_0) + Ixz*Iyz*Kq*gamma3_0*tau3_0*cos(gamma3_0) + Ixy*Izz*Kq*gamma2_0*tau2_0*cos(gamma2_0) + Ixy*Izz*Kq*gamma3_0*tau3_0*cos(gamma3_0) + Iyy*Izz*Kq*gamma1_0*tau1_0*cos(gamma1_0) - Ixz*Iyz*Kq*eta1_0*tau1_0*cos(eta1_0)*cos(gamma1_0) - Ixy*Izz*Kq*eta1_0*tau1_0*cos(eta1_0)*cos(gamma1_0) - Iyy*Izz*Kq*eta2_0*tau2_0*cos(eta2_0)*cos(gamma2_0) - Iyy*Izz*Kq*eta3_0*tau3_0*cos(eta3_0)*cos(gamma3_0) - Ixy*Iyz*Kq*eta1_0*tau1_0*cos(gamma1_0)*sin(eta1_0) - Ixz*Iyy*Kq*eta1_0*tau1_0*cos(gamma1_0)*sin(eta1_0) + Ixy*Iyz*Kq*eta2_0*tau2_0*cos(gamma2_0)*sin(eta2_0) + Ixz*Iyy*Kq*eta2_0*tau2_0*cos(gamma2_0)*sin(eta2_0) + Ixy*Iyz*Kq*eta3_0*tau3_0*cos(gamma3_0)*sin(eta3_0) + Ixz*Iyy*Kq*eta3_0*tau3_0*cos(gamma3_0)*sin(eta3_0) - Ixy*Iyz*Kq*gamma1_0*tau1_0*cos(eta1_0)*sin(gamma1_0) - Ixz*Iyy*Kq*gamma1_0*tau1_0*cos(eta1_0)*sin(gamma1_0) + Ixy*Iyz*Kq*gamma2_0*tau2_0*cos(eta2_0)*sin(gamma2_0) + Ixz*Iyy*Kq*gamma2_0*tau2_0*cos(eta2_0)*sin(gamma2_0) + Ixy*Iyz*Kq*gamma3_0*tau3_0*cos(eta3_0)*sin(gamma3_0) + Ixz*Iyy*Kq*gamma3_0*tau3_0*cos(eta3_0)*sin(gamma3_0) + Ixz*Iyz*Kq*gamma1_0*tau1_0*sin(eta1_0)*sin(gamma1_0) + Ixy*Izz*Kq*gamma1_0*tau1_0*sin(eta1_0)*sin(gamma1_0) + Iyy*Izz*Kq*gamma2_0*tau2_0*sin(eta2_0)*sin(gamma2_0) + Iyy*Izz*Kq*gamma3_0*tau3_0*sin(eta3_0)*sin(gamma3_0))/(Izz*Ixy^2 + 2*Ixy*Ixz*Iyz + Iyy*Ixz^2 + Ixx*Iyz^2 - Ixx*Iyy*Izz);
                                                                                                                                                                                                                                                                                                                                                                                                                                                                                                                                                                                                                                                                                                                                                                                                                                                                                                                                                                                                                                                                                                                                                                                                                                                                                                                                                                                                                                                                                                                                                                                                                                                                                                                                                                                                                                                                                                                                                                                                                                                                                                                                                                                                                                                                                                                                                                                                                                                                                                                                                                                                                                                                                                                                                                                                                                                                                                                                                                                                                                                                                                                                                                                                                                                                                                                                                                                                                                                                                                                                                                                                                                                                                                                                                                                                                                                                                                                                                                                                                                                                                                                                                                                                                                                                                                                                                                                                                                                                                                                                                                                                                                                                                                                                                                                                                                                                                                                                                                                                                                                                                                                                                                                                                                                                                                                                                                                                                                                                                                                                                                                                                                                                                           -(Ixz^3*P^2 - Ixz^3*R^2 + Ixy^2*Ixz*P^2 - Ixy^2*Ixz*Q^2 + Ixz*Iyz^2*Q^2 - Ixz*Iyz^2*R^2 + Ixx*Ixy*Iyz*P^2 - Ixx*Ixz*Izz*P^2 - Ixx*Ixy*Iyz*Q^2 + Ixy*Iyz*Izz*Q^2 + Ixx*Ixz*Izz*R^2 - Ixy*Iyz*Izz*R^2 + Ixx^2*Iyz*P*Q + 2*Ixz^2*Iyz*P*Q + Ixx*Ixz^2*P*R + Ixx*Iyz^2*P*R + Ixx*Izz^2*P*R - Ixx^2*Izz*P*R - Ixy^2*Izz*P*R - Ixz^2*Izz*P*R - 2*Ixy*Ixz^2*Q*R - Ixy*Izz^2*Q*R + Ixx*Ixy*Ixz*P*Q - Ixy*Ixz*Iyy*P*Q - Ixx*Iyy*Iyz*P*Q + Ixy*Ixz*Izz*P*Q - Ixx*Iyz*Izz*P*Q - Ixx*Ixz*Iyz*Q*R + Ixx*Ixy*Izz*Q*R + Ixz*Iyy*Iyz*Q*R + Ixy*Iyy*Izz*Q*R - Ixz*Iyz*Izz*Q*R - Ixz^2*Kq*gamma2_0*tau2_0*cos(gamma2_0) - Ixz^2*Kq*gamma3_0*tau3_0*cos(gamma3_0) + Ixz^2*Kq*eta1_0*tau1_0*cos(eta1_0)*cos(gamma1_0) - Ixz^2*Kq*gamma1_0*tau1_0*sin(eta1_0)*sin(gamma1_0) + Ixz*Iyz*Kq*gamma1_0*tau1_0*cos(gamma1_0) + Ixx*Izz*Kq*gamma2_0*tau2_0*cos(gamma2_0) + Ixx*Izz*Kq*gamma3_0*tau3_0*cos(gamma3_0) + Ixy*Izz*Kq*gamma1_0*tau1_0*cos(gamma1_0) - Ixz*Iyz*Kq*eta2_0*tau2_0*cos(eta2_0)*cos(gamma2_0) - Ixz*Iyz*Kq*eta3_0*tau3_0*cos(eta3_0)*cos(gamma3_0) - Ixx*Izz*Kq*eta1_0*tau1_0*cos(eta1_0)*cos(gamma1_0) - Ixy*Izz*Kq*eta2_0*tau2_0*cos(eta2_0)*cos(gamma2_0) - Ixy*Izz*Kq*eta3_0*tau3_0*cos(eta3_0)*cos(gamma3_0) - Ixy*Ixz*Kq*eta1_0*tau1_0*cos(gamma1_0)*sin(eta1_0) + Ixy*Ixz*Kq*eta2_0*tau2_0*cos(gamma2_0)*sin(eta2_0) + Ixy*Ixz*Kq*eta3_0*tau3_0*cos(gamma3_0)*sin(eta3_0) - Ixx*Iyz*Kq*eta1_0*tau1_0*cos(gamma1_0)*sin(eta1_0) + Ixx*Iyz*Kq*eta2_0*tau2_0*cos(gamma2_0)*sin(eta2_0) + Ixx*Iyz*Kq*eta3_0*tau3_0*cos(gamma3_0)*sin(eta3_0) - Ixy*Ixz*Kq*gamma1_0*tau1_0*cos(eta1_0)*sin(gamma1_0) + Ixy*Ixz*Kq*gamma2_0*tau2_0*cos(eta2_0)*sin(gamma2_0) + Ixy*Ixz*Kq*gamma3_0*tau3_0*cos(eta3_0)*sin(gamma3_0) - Ixx*Iyz*Kq*gamma1_0*tau1_0*cos(eta1_0)*sin(gamma1_0) + Ixx*Iyz*Kq*gamma2_0*tau2_0*cos(eta2_0)*sin(gamma2_0) + Ixx*Iyz*Kq*gamma3_0*tau3_0*cos(eta3_0)*sin(gamma3_0) + Ixz*Iyz*Kq*gamma2_0*tau2_0*sin(eta2_0)*sin(gamma2_0) + Ixz*Iyz*Kq*gamma3_0*tau3_0*sin(eta3_0)*sin(gamma3_0) + Ixx*Izz*Kq*gamma1_0*tau1_0*sin(eta1_0)*sin(gamma1_0) + Ixy*Izz*Kq*gamma2_0*tau2_0*sin(eta2_0)*sin(gamma2_0) + Ixy*Izz*Kq*gamma3_0*tau3_0*sin(eta3_0)*sin(gamma3_0))/(Izz*Ixy^2 + 2*Ixy*Ixz*Iyz + Iyy*Ixz^2 + Ixx*Iyz^2 - Ixx*Iyy*Izz);
                                                                                                                                                                                                                                                                                                                                                                                                                                                                                                                                                                                                                                                                                                                                                                                                                                                                                                                                                                                                                                                                                                                                                                                                                                                                                                                                                                                                                                                                                                                                                                                                                                                                                                                                                                                                                                                                                                                                                                                                                                                                                                                                                                                                                                                                                                                                                                                                                                                                                                                                                                                                                                                                                                                                                                                                                                                                                                                                                                                                                                                                                                                                                                                                                                                                                                                                                                                                                                                                                                                                                                                                                                                                                                                                                                                                                                                                                                                                                                                                                                                                                                                                                                                                                                                                                                                                                                                                                                                                                                                                                                                                                                                                                                                                                                                                                                                                                                                                                                                                                                                                                                                                                                                                                                                                                                                                                                                                                                                                                                                                                                                                                                                                                               -(Ixy^3*Q^2 - Ixy^3*P^2 - Ixy*Ixz^2*P^2 + Ixy*Iyz^2*Q^2 + Ixy*Ixz^2*R^2 - Ixy*Iyz^2*R^2 + Ixx*Ixy*Iyy*P^2 - Ixx*Ixz*Iyz*P^2 - Ixx*Ixy*Iyy*Q^2 + Ixz*Iyy*Iyz*Q^2 + Ixx*Ixz*Iyz*R^2 - Ixz*Iyy*Iyz*R^2 - Ixx*Ixy^2*P*Q - Ixx*Iyy^2*P*Q + Ixx^2*Iyy*P*Q - Ixx*Iyz^2*P*Q + Ixy^2*Iyy*P*Q + Ixz^2*Iyy*P*Q - Ixx^2*Iyz*P*R - 2*Ixy^2*Iyz*P*R + 2*Ixy^2*Ixz*Q*R + Ixz*Iyy^2*Q*R - Ixx*Ixy*Ixz*P*R - Ixy*Ixz*Iyy*P*R + Ixx*Iyy*Iyz*P*R + Ixy*Ixz*Izz*P*R + Ixx*Iyz*Izz*P*R + Ixx*Ixy*Iyz*Q*R - Ixx*Ixz*Iyy*Q*R + Ixy*Iyy*Iyz*Q*R - Ixy*Iyz*Izz*Q*R - Ixz*Iyy*Izz*Q*R + Ixy^2*Kq*eta1_0*tau1_0*cos(gamma1_0)*sin(eta1_0) - Ixy^2*Kq*eta2_0*tau2_0*cos(gamma2_0)*sin(eta2_0) - Ixy^2*Kq*eta3_0*tau3_0*cos(gamma3_0)*sin(eta3_0) + Ixy^2*Kq*gamma1_0*tau1_0*cos(eta1_0)*sin(gamma1_0) - Ixy^2*Kq*gamma2_0*tau2_0*cos(eta2_0)*sin(gamma2_0) - Ixy^2*Kq*gamma3_0*tau3_0*cos(eta3_0)*sin(gamma3_0) + Ixy*Ixz*Kq*gamma2_0*tau2_0*cos(gamma2_0) + Ixy*Ixz*Kq*gamma3_0*tau3_0*cos(gamma3_0) + Ixx*Iyz*Kq*gamma2_0*tau2_0*cos(gamma2_0) + Ixx*Iyz*Kq*gamma3_0*tau3_0*cos(gamma3_0) + Ixy*Iyz*Kq*gamma1_0*tau1_0*cos(gamma1_0) + Ixz*Iyy*Kq*gamma1_0*tau1_0*cos(gamma1_0) - Ixy*Ixz*Kq*eta1_0*tau1_0*cos(eta1_0)*cos(gamma1_0) - Ixx*Iyz*Kq*eta1_0*tau1_0*cos(eta1_0)*cos(gamma1_0) - Ixy*Iyz*Kq*eta2_0*tau2_0*cos(eta2_0)*cos(gamma2_0) - Ixz*Iyy*Kq*eta2_0*tau2_0*cos(eta2_0)*cos(gamma2_0) - Ixy*Iyz*Kq*eta3_0*tau3_0*cos(eta3_0)*cos(gamma3_0) - Ixz*Iyy*Kq*eta3_0*tau3_0*cos(eta3_0)*cos(gamma3_0) - Ixx*Iyy*Kq*eta1_0*tau1_0*cos(gamma1_0)*sin(eta1_0) + Ixx*Iyy*Kq*eta2_0*tau2_0*cos(gamma2_0)*sin(eta2_0) + Ixx*Iyy*Kq*eta3_0*tau3_0*cos(gamma3_0)*sin(eta3_0) - Ixx*Iyy*Kq*gamma1_0*tau1_0*cos(eta1_0)*sin(gamma1_0) + Ixx*Iyy*Kq*gamma2_0*tau2_0*cos(eta2_0)*sin(gamma2_0) + Ixx*Iyy*Kq*gamma3_0*tau3_0*cos(eta3_0)*sin(gamma3_0) + Ixy*Ixz*Kq*gamma1_0*tau1_0*sin(eta1_0)*sin(gamma1_0) + Ixx*Iyz*Kq*gamma1_0*tau1_0*sin(eta1_0)*sin(gamma1_0) + Ixy*Iyz*Kq*gamma2_0*tau2_0*sin(eta2_0)*sin(gamma2_0) + Ixz*Iyy*Kq*gamma2_0*tau2_0*sin(eta2_0)*sin(gamma2_0) + Ixy*Iyz*Kq*gamma3_0*tau3_0*sin(eta3_0)*sin(gamma3_0) + Ixz*Iyy*Kq*gamma3_0*tau3_0*sin(eta3_0)*sin(gamma3_0))/(Izz*Ixy^2 + 2*Ixy*Ixz*Iyz + Iyy*Ixz^2 + Ixx*Iyz^2 - Ixx*Iyy*Izz)];
